simulink model "mdltop"  (R2022b)
settings: Solver=FixedStepAuto  StartTime=0.0  StopTime=.18  FixedStep=.1  RelTol=1e-3
settings Model: Creator=hp_desktop  LastModifiedBy=hp_desktop
settings OptimizationCC: OptimizeBlockIOStorage=off

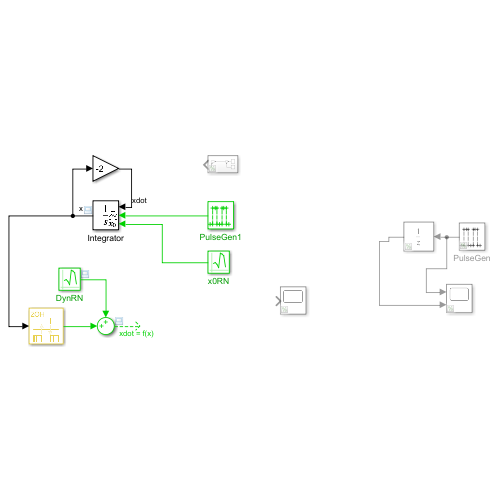
[thumbnail: Simulink's stored preview of the top-level diagram]
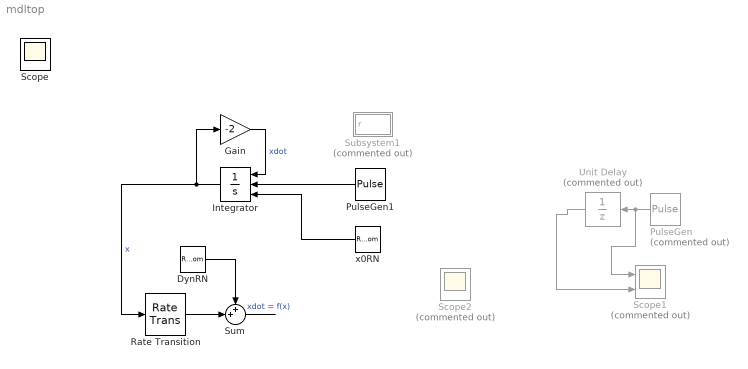
== system mdltop ==
  DynRN : RandomNumber  SampleTime=.06
  Gain : Gain  Gain=-2
  Integrator : Integrator  ExternalReset=either  InitialConditionSource=external
  PulseGen : DiscretePulseGenerator  Commented=on  SampleTime=.04
  PulseGen1 : DiscretePulseGenerator  SampleTime=.06
  Rate Transition : RateTransition  OutPortSampleTime=.06
  Scope1 : Scope  Commented=on  NumInputPorts=2
  Scope2 : Scope  Commented=on
  Subsystem1 : Subsystem  Commented=on
  Sum : Sum  Inputs=++|
  Unit Delay : UnitDelay  Commented=on  InitialCondition=1  SampleTime=.01  HasFrameUpgradeWarning=on
  x0RN : RandomNumber  SampleTime=.06
  Scope : Scope
  wires:
  DynRN/1 -> Sum/1
  PulseGen/1 -> Unit Delay/1, Scope1/1
  Unit Delay/1 -> Scope1/2
  PulseGen1/1 -> Integrator/2
  Integrator/1 -> Rate Transition/1, Gain/1  "x"
  Gain/1 -> Integrator/1  "xdot"
  Rate Transition/1 -> Sum/2
  Sum/1 -> ?  "xdot = f(x)"
  x0RN/1 -> Integrator/3

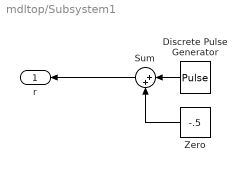
== system mdltop/Subsystem1 ==
  Discrete Pulse Generator : DiscretePulseGenerator  SampleTime=.1
  Sum : Sum  Inputs=|++
  Zero : Constant  Value=-.5  OutDataTypeStr=Inherit: Inherit via back propagation
  r : Outport
  wires:
  Sum/1 -> r/1
  Discrete Pulse Generator/1 -> Sum/1
  Zero/1 -> Sum/2
